simulink library "vmc"  (R2021b)
settings: Solver=VariableStepAuto  StartTime=0.0  StopTime=10.0  RelTol=1e-3
undefined symbols (not defined in the file or in its folder): AVMC_ACCDeltaTqIGain_X_kph, AVMC_ACCDeltaTqIGain_Y_mps2, AVMC_ACCDeltaTqIGainP2_X_kph, AVMC_ACCDeltaTqIGainP2_Y_mps2, AVMC_ACCDeltaTqPGain_X_kph, AVMC_ACCDeltaTqPGain_Y_kph, AVMC_ACCDeltaTqPGainP2_X_kph, AVMC_ACCDeltaTqPGainP2_Y_kph, AVMC_ACCLongSteadyCtrl_X_kph, AVMC_CCAccelCMD_X_kph, AVMC_CCAccelCMD_Y_kph, AVMC_CCDeltaTqIGain_X_kph, AVMC_CCDeltaTqIGain_Y_mps2, AVMC_CCDeltaTqPGain_X_kph, AVMC_CCDeltaTqPGain_Y_kph, AVMC_CCLongSteadyCtrl_X_kph, AVMC_DISCDeltaTqIGainP2_X_kph, AVMC_DISCDeltaTqIGainP2_Y_mps2, AVMC_ESCRegenOut_X_kph, AVMC_ESCRegenOut_Y_Deg, AVMC_ESCRegenOutEnSpd_X_Deg, AVMC_LatESCRegenOut_X_kph, AVMC_LatESCRegenOut_Y_Deg, AVMC_LongAccDeadZone_X_kph, AVMC_LongAccDeadZoneP2_X_kph, AVMC_LongAccFiltTs_X_Gps, AVMC_LongAccFiltTsP2_X_Gps, AVMC_MCPresBaseTq_X_bar, AVMC_MSAAccelCMD_X_kph, AVMC_MSAAccelCMD_Y_kph, AVMC_MSADeltaTqIGain_X_kph, AVMC_MSADeltaTqIGain_Y_mps2, AVMC_MSADeltaTqPGain_X_kph, AVMC_MSADeltaTqPGain_Y_kph, AVMC_MSALongSteadyCtrl_X_kph, AVMC_MSAPedalOvrd_X_kph, AVMC_MSASpdBand_X_kph, AVMC_OPDDisSlideRate_X_Deg, AVMC_RDCDetectTime_X_kph, AVMC_RDCDetectTime_Y_pct, AVMC_RDCEnSlideRate_X_Deg, AVMC_StESCYaw_X_kph, AVMC_StESCYaw_Y_Deg, AVMC_StESCYawCom_X_kph, AVMC_StESCYawCom_Y_Gps, AVMC_TMSpdBaseTq_X_rpm, C_TASK_10MS_S, C_TASK_5MS_S, DEG2RAD, Discrete, ENUM_ADASACCSTA_ACTIVE, ENUM_ADASACCSTA_OVERRIDE, ENUM_ADASACCSTA_STANDBY, ENUM_ADASMSASTA_ACTIVE, ENUM_ADASMSASTA_ERROR, ENUM_ADASMSASTA_OFF, ENUM_ADASMSASTA_OVERSPEED, ENUM_ADASMSASTA_STANDBY, ENUM_ADASMSASTA_UNDERSPEED, ENUM_ADASMSASTA_UNLIMIT ... (+254)
libraries: hcu_lib x57, simulink x49, ctrlSharedLib x6, simulink_extras x1
(part 2 of 9)

== system vmc/VMC/APS function ==
  VTQD_ExternalTqAllow_flg : Inport
  VTQD_ExtShiftAllow_flg : Inport  Port=2
  VTQD_ExtDoorAllow_flg : Inport  Port=3
  VTQD_GearActualPosn_enum : Inport  Port=4
  VINP_APSStaSys_enum : Inport  Port=5
  VINP_APSVMCReqA_flg : Inport  Port=6
  VINP_APSShiftPosnReq_enum : Inport  Port=7
  VINP_APSSpeedCMD_kph : Inport  Port=8
  VINP_CAASVMCReqA_flg : Inport  Port=9
  task_time_s : Inport  Port=10
  BTQD_outputs : Inport  Port=11  OutDataTypeStr=Bus: BTQD_outputs
  VINP_SCPSystemMode_enum : Inport  Port=12
  VVMC_ADASActive_flg : Inport  Port=13
  BINP_APM_outputs : Inport  Port=14  OutDataTypeStr=Bus: BINP_APM_outputs
  VINP_VehSpeed_kph : Inport  Port=15
  VVMC_CruzActive_flg : Inport  Port=16
  VINP_ADASACCSta_enum : Inport  Port=17
  VINP_MCPressure_bar : Inport  Port=18
  VINP_BrkSwSta_flg : Inport  Port=19
  VINP_BrkPedalPos_pct : Inport  Port=20
  VVMC_AllowSetSpd_flg : Inport  Port=21
  AND : Logic  Inputs=4  AllPortsSameDT=off  OutDataTypeStr=boolean
  AND1 : Logic  Operator=OR  AllPortsSameDT=off  OutDataTypeStr=boolean
  AND2 : Logic  Inputs=4  AllPortsSameDT=off  OutDataTypeStr=boolean
  Bus Selector3 : BusSelector  OutputSignals=VTQD_APSDecReqA_flg
  CAAS HandShake : Subsystem
  Command Determination : Subsystem
  Constant1 : Constant  Value=ENUM_ADASACCSTA_ACTIVE
  Constant2 : Constant  Value=ENUM_ADASACCSTA_STANDBY
  Constant3 : Constant  Value=KVMC_APSACCSetTest_flg
  Constant4 : Constant  Value=KVMC_APSAllowSetACCMCP_bar
  Constant5 : Constant  Value=ZERO_FLOAT
  Constant6 : Constant  Value=TRUE
  Constant7 : Constant  Value=KVMC_APSAllowSetACCPosn_pct
  Data Type Conversion : DataTypeConversion  OutDataTypeStr=uint8
  Hand Shake : Subsystem
  NOT : Logic  Operator=NOT  AllPortsSameDT=off  OutDataTypeStr=boolean
  NOT1 : Logic  Operator=NOT  AllPortsSameDT=off  OutDataTypeStr=boolean
  Relational Operator : RelationalOperator  Operator===  OutDataTypeStr=boolean  RndMeth=Simplest
  Relational Operator1 : RelationalOperator  Operator===  OutDataTypeStr=boolean  RndMeth=Simplest
  Relational Operator2 : RelationalOperator  Operator=>  OutDataTypeStr=boolean  RndMeth=Simplest
  Relational Operator3 : RelationalOperator  Operator=>  OutDataTypeStr=boolean  RndMeth=Simplest
  Relational Operator4 : RelationalOperator  Operator=>  OutDataTypeStr=boolean  RndMeth=Simplest
  SR_Latch2 : hcu_lib/Basic_Blocks/SR_Latch
  Signal Rounting : Subsystem
  Switch : Switch  Criteria=u2 > Threshold
  VVMC_APSCtrlAvail_flg : Outport
  VVMC_APSActive_flg : Outport  Port=2
  VVMC_APSSpeedCMD_kph : Outport  Port=3
  VVMC_APSShiftPosnReq_enum : Outport  Port=4
  VVMC_APSStaSys_enum : Outport  Port=5
  VVMC_APSDecReqA_flg : Outport  Port=6
  VVMC_APSDecReq_mps2 : Outport  Port=7
  VVMC_APSReq_enum : Outport  Port=8
  VVMC_CAASCtrlAvail_flg : Outport  Port=9
  VVMC_CAASActive_flg : Outport  Port=10
  wires:
  Command Determination/2(VVMC_APSShiftPosnReq_enum) -> VVMC_APSShiftPosnReq_enum/1
  Command Determination/1(VVMC_APSSpeedCMD_kph) -> VVMC_APSSpeedCMD_kph/1
  [VINP_APSSpeedCMD_kph] -> Command Determination/4(VINP_APSSpeedCMD_kph)
  [VINP_APSShiftPosnReq_enum] -> Command Determination/3(VINP_APSShiftPosnReq_enum)
  [VINP_APSStaSys_enum] -> Command Determination/2(VINP_APSStaSys_enum)
  [VVMC_APSActive_flg] -> Command Determination/1(VVMC_APSActive_flg)
  [VTQD_ExtShiftAllow_flg] -> Hand Shake/3(VTQD_ExtShiftAllow_flg)
  [VTQD_ExternalTqAllow_flg] -> Hand Shake/2(VTQD_ExternalTqAllow_flg)
  [task_time_s] -> Hand Shake/1(task_time_s)
  task_time_s/1 -> [task_time_s]
  VINP_APSSpeedCMD_kph/1 -> [VINP_APSSpeedCMD_kph]
  VINP_APSShiftPosnReq_enum/1 -> [VINP_APSShiftPosnReq_enum]
  VINP_APSVMCReqA_flg/1 -> [VINP_APSVMCReqA_flg]
  VINP_APSStaSys_enum/1 -> [VINP_APSStaSys_enum]
  VVMC_ADASActive_flg/1 -> [VVMC_ADASActive_flg]
  BTQD_outputs/1 -> [BTQD_outputs]
  [VVMC_APSActive_flg] -> Signal Rounting/3(VVMC_APSActive_flg)
  [VVMC_ADASActive_flg] -> Signal Rounting/4(VVMC_ADASActive_flg)
  [BTQD_outputs] -> Signal Rounting/2(BTQD_outputs)
  Signal Rounting/1(VVMC_APSStaSys_enum) -> VVMC_APSStaSys_enum/1
  Signal Rounting/4(VVMC_APSReq_enum) -> VVMC_APSReq_enum/1
  Signal Rounting/3(VVMC_APSDecReq_mps2) -> VVMC_APSDecReq_mps2/1
  Signal Rounting/2(VVMC_APSDecReqA_flg) -> VVMC_APSDecReqA_flg/1
  VTQD_ExtDoorAllow_flg/1 -> [VTQD_ExtDoorAllow_flg]
  VTQD_ExternalTqAllow_flg/1 -> [VTQD_ExternalTqAllow_flg]
  VTQD_ExtShiftAllow_flg/1 -> [VTQD_ExtShiftAllow_flg]
  VINP_SCPSystemMode_enum/1 -> Data Type Conversion/1
  [VTQD_ExtDoorAllow_flg] -> Hand Shake/6(VTQD_ExtDoorAllow_flg)
  [BINP_APM_outputs] -> Signal Rounting/5(BINP_APM_outputs)
  [VINP_APSVMCReqA_flg] -> Hand Shake/4(VINP_APSVMCReqA_flg)
  [VINP_APSStaSys_enum] -> Hand Shake/5(VINP_APSStaSys_enum)
  BINP_APM_outputs/1 -> [BINP_APM_outputs]
  VTQD_GearActualPosn_enum/1 -> [VTQD_GearActualPosn_enum]
  [VINP_SCPSystemMode_enum] -> Signal Rounting/1(VINP_SCPSystemMode_enum)
  [VTQD_GearActualPosn_enum] -> Signal Rounting/6(VTQD_GearActualPosn_enum)
  Data Type Conversion/1 -> [VINP_SCPSystemMode_enum]
  VINP_CAASVMCReqA_flg/1 -> [VINP_CAASVMCReqA_flg]
  [VVMC_CAASActive_flg] -> Signal Rounting/7(VVMC_CAASActive_flg)
  [task_time_s] -> CAAS HandShake/4(task_time_s)
  [VVMC_CruzActive_flg] -> CAAS HandShake/3(VVMC_CruzActive_flg)
  CAAS HandShake/2(VVMC_CAASActive_flg) -> VVMC_CAASActive_flg/1, [VVMC_CAASActive_flg]
  [VINP_VehSpeed_kph] -> CAAS HandShake/1(VINP_VehSpeed_kph)
  [VVMC_ADASActive_flg] -> CAAS HandShake/2(VVMC_ADASActive_flg)
  CAAS HandShake/1(VVMC_CAASCtrlAvail_flg) -> VVMC_CAASCtrlAvail_flg/1
  [VINP_CAASVMCReqA_flg] -> CAAS HandShake/5(VINP_CAASVMCReqA_flg)
  VINP_VehSpeed_kph/1 -> [VINP_VehSpeed_kph]
  VVMC_CruzActive_flg/1 -> [VVMC_CruzActive_flg]
  Hand Shake/1(VVMC_APSCtrlAvail_flg) -> VVMC_APSCtrlAvail_flg/1
  Hand Shake/2(VVMC_APSActive_flg) -> [VVMC_APSActive_flg], VVMC_APSActive_flg/1
  Relational Operator4/1 -> AND2/4
  Constant2/1 -> Relational Operator/2
  VINP_BrkPedalPos_pct/1 -> Relational Operator4/1
  Constant5/1 -> Relational Operator3/2
  [BTQD_outputs] -> Bus Selector3/1
  AND/1 -> SR_Latch2/1
  Relational Operator2/1 -> AND2/2
  Constant6/1 -> Switch/3
  VINP_MCPressure_bar/1 -> Relational Operator2/1
  AND2/1 -> AND/3
  [VINP_BrkSwSta_flg] -> NOT/1
  VINP_BrkSwSta_flg/1 -> [VINP_BrkSwSta_flg], AND2/1
  [VINP_VehSpeed_kph] -> Relational Operator3/1
  Constant3/1 -> AND/4
  NOT1/1 -> AND2/3
  Relational Operator3/1 -> NOT1/1
  SR_Latch2/1 -> Switch/1  "VVMC_SetACCDisableAPS_flg"
  NOT/1 -> AND1/2
  Constant7/1 -> Relational Operator4/2
  VINP_ADASACCSta_enum/1 -> [VINP_ADASACCSta_enum], Relational Operator/1
  Switch/1 -> [VVMC_SetACCDisableAPS_flg]
  Constant1/1 -> Relational Operator1/2
  Constant4/1 -> Relational Operator2/2
  Relational Operator/1 -> AND/1
  Relational Operator1/1 -> AND1/1
  AND1/1 -> SR_Latch2/2
  VVMC_AllowSetSpd_flg/1 -> AND/2
  [VINP_ADASACCSta_enum] -> Relational Operator1/1
  Bus Selector3/1 -> Switch/2  "<VTQD_APSDecReqA_flg>"
  [VVMC_SetACCDisableAPS_flg] -> Signal Rounting/8(VVMC_SetACCDisableAPS_flg)

== system vmc/VMC/CruiseControlFunction ==
  VTQD_ExternalTqAllow_flg : Inport
  VTQD_DriverWhlTqDem_Nm : Inport  Port=2
  VTQD_LowIdleAccPedal_flg : Inport  Port=3
  VTQD_GearActualPosn_enum : Inport  Port=4
  VTQD_ExtDoorAllow_flg : Inport  Port=5
  VINP_ZoneSpdCrlMode_enum : Inport  Port=6
  VINP_SetSpd_kph : Inport  Port=7
  VINP_SWCResUpSta_flg : Inport  Port=8
  VINP_SWCSetdownSta_flg : Inport  Port=9
  VINP_SWCCANCELSta_flg : Inport  Port=10
  VINP_BrakeSWGPIO_flg : Inport  Port=11
  VINP_BrkSwSta_flg : Inport  Port=12
  VINP_VehSpeed_kph : Inport  Port=13
  VINP_BrkPedalPos_pct : Inport  Port=14
  VVMC_LongAcc_Gps : Inport  Port=15
  VVMC_CalMeterSpeed_kph : Inport  Port=16
  CCActiveDetermination : Subsystem
  CCDemandTorqueCalculation : Subsystem
  CCTorqueSourceDetermination : Subsystem
  Data Type Conversion : DataTypeConversion  OutDataTypeStr=uint8
  VVMC_CCCtrlSta_enum : Outport
  VVMC_CCSpdWar_flg : Outport  Port=2
  VVMC_CruzWhlTqReq_N m : Outport  Port=3
  VVMC_CruzActive_flg : Outport  Port=4
  VVMC_CCPedalOvrd_flg : Outport  Port=5
  wires:
  [VVMC_CruzWhlTqReq_Nm] -> VVMC_CruzWhlTqReq_N m/1
  VINP_SWCResUpSta_flg/1 -> [VINP_SWCResUpSta_flg]
  VINP_SWCCANCELSta_flg/1 -> [VINP_SWCCANCELSta_flg]
  VTQD_DriverWhlTqDem_Nm/1 -> [VTQD_DriverWhlTqDem_Nm]
  VINP_ZoneSpdCrlMode_enum/1 -> [VINP_ZoneSpdCrlMode_enum]
  VINP_VehSpeed_kph/1 -> [VINP_VehSpeed_kph]
  VTQD_LowIdleAccPedal_flg/1 -> [VTQD_LowIdleAccPedal_flg]
  [VVMC_CCCtrlSta_enum] -> VVMC_CCCtrlSta_enum/1
  [VVMC_CCSpdWar_flg] -> VVMC_CCSpdWar_flg/1
  [VVMC_CruzActive_flg] -> VVMC_CruzActive_flg/1
  VINP_SWCSetdownSta_flg/1 -> [VINP_SWCSetdownSta_flg]
  VVMC_LongAcc_Gps/1 -> [VVMC_LongAcc_Gps]
  VTQD_ExternalTqAllow_flg/1 -> [VTQD_ExternalTqAllow_flg]
  VINP_BrkSwSta_flg/1 -> [VINP_BrkSwSta_flg]
  VINP_SetSpd_kph/1 -> [VINP_SetSpd_kph]
  [VVMC_CCPedalOvrd_flg] -> VVMC_CCPedalOvrd_flg/1
  VINP_BrakeSWGPIO_flg/1 -> [VINP_BrakeSWGPIO_flg]
  CCTorqueSourceDetermination/2(VVMC_CCPedalOvrd_flg) -> [VVMC_CCPedalOvrd_flg]
  CCTorqueSourceDetermination/1(VVMC_CruzWhlTqReq_Nm) -> [VVMC_CruzWhlTqReq_Nm]
  [VTQD_DriverWhlTqDem_Nm] -> CCTorqueSourceDetermination/1(VTQD_DriverWhlTqDem_Nm)
  [VTQD_LowIdleAccPedal_flg] -> CCTorqueSourceDetermination/4(VTQD_LowIdleAccPedal_flg)
  [VVMC_CruzActive_flg] -> CCTorqueSourceDetermination/3(VVMC_CruzActive_flg)
  [VVMC_CruzWhlTqCal_Nm] -> CCTorqueSourceDetermination/2(VVMC_CruzWhlTqCal_Nm)
  [VINP_VehSpeed_kph] -> CCDemandTorqueCalculation/2(VINP_VehSpeed_kph)
  [VVMC_CCPedalOvrd_flg] -> CCDemandTorqueCalculation/6(VVMC_CCPedalOvrd_flg)
  [VINP_SetSpd_kph] -> CCDemandTorqueCalculation/1(VINP_SetSpd_kph)
  [VVMC_CruzActive_flg] -> CCDemandTorqueCalculation/3(VVMC_CruzActive_flg)
  CCDemandTorqueCalculation/1(VVMC_CruzWhlTqCal_Nm) -> [VVMC_CruzWhlTqCal_Nm]
  [VTQD_DriverWhlTqDem_Nm] -> CCDemandTorqueCalculation/4(VTQD_DriverWhlTqDem_Nm)
  [VVMC_LongAcc_Gps] -> CCDemandTorqueCalculation/5(VVMC_LongAcc_Gps)
  [VINP_SWCSetdownSta_flg] -> CCActiveDetermination/3(VINP_SWCSetdownSta_flg)
  [VINP_SetSpd_kph] -> Data Type Conversion/1
  [VVMC_CCPedalOvrd_flg] -> CCActiveDetermination/10(VVMC_CCPedalOvrd_flg)
  [VINP_SWCCANCELSta_flg] -> CCActiveDetermination/8(VINP_SWCCANCELSta_flg)
  CCActiveDetermination/3(VVMC_CruzActive_flg) -> [VVMC_CruzActive_flg]
  CCActiveDetermination/1(VVMC_CCCtrlSta_enum) -> [VVMC_CCCtrlSta_enum]
  [VTQD_ExternalTqAllow_flg] -> CCActiveDetermination/2(VTQD_ExternalTqAllow_flg)
  [VINP_ZoneSpdCrlMode_enum] -> CCActiveDetermination/1(VINP_ZoneSpdCrlMode_enum)
  [VINP_VehSpeed_kph] -> CCActiveDetermination/5(VINP_VehSpeed_kph)
  [VINP_BrakeSWGPIO_flg] -> CCActiveDetermination/7(VINP_BrakeSWGPIO_flg)
  [VINP_SWCResUpSta_flg] -> CCActiveDetermination/4(VINP_SWCResUpSta_flg)
  [VINP_BrkSwSta_flg] -> CCActiveDetermination/9(VINP_BrkSwSta_flg)
  CCActiveDetermination/2(VVMC_CCSpdWar_flg) -> [VVMC_CCSpdWar_flg]
  VTQD_GearActualPosn_enum/1 -> [VTQD_GearActualPosn_enum]
  [VTQD_GearActualPosn_enum] -> CCActiveDetermination/11(VTQD_GearActualPosn_enum)
  VVMC_CalMeterSpeed_kph/1 -> [VVMC_CalMeterSpeed_kph]
  [VVMC_CalMeterSpeed_kph] -> CCDemandTorqueCalculation/7(VVMC_CalMeterSpeed_kph)
  VINP_BrkPedalPos_pct/1 -> [VINP_BrkPedalPos_pct]
  [VINP_BrkPedalPos_pct] -> CCActiveDetermination/12(VINP_BrkPedalPos_pct)
  Data Type Conversion/1 -> CCActiveDetermination/6(VINP_SetSpd_kph)
  VTQD_ExtDoorAllow_flg/1 -> [VTQD_ExtDoorAllow_flg]
  [VTQD_ExtDoorAllow_flg] -> CCActiveDetermination/13(VTQD_ExtDoorAllow_flg)
  [VVMC_CalMeterSpeed_kph] -> CCActiveDetermination/14(VVMC_CalMeterSpeed_kph)

== system vmc/VMC/IMU ==
  VINP_MemOffsetGyroX_raw16 : Inport
  VINP_MemOffsetGyroY_raw16 : Inport  Port=2
  VINP_MemOffsetGyroZ_raw16 : Inport  Port=3
  VINP_MemOffsetAccX_raw16 : Inport  Port=4
  VINP_MemOffsetAccY_raw16 : Inport  Port=5
  VINP_MemOffsetAccZ_raw16 : Inport  Port=6
  VINP_SensingGyroX_raw16 : Inport  Port=7
  VINP_SensingGyroY_raw16 : Inport  Port=8
  VINP_SensingGyroZ_raw16 : Inport  Port=9
  VINP_SensingAccX_raw16 : Inport  Port=10
  VINP_SensingAccY_raw16 : Inport  Port=11
  VINP_SensingAccZ_raw16 : Inport  Port=12
  task_time_s : Inport  Port=13
  Constant : Constant  Value=KVMC_IMUEnaCmd_flg
  IMU memorized offset result : Subsystem
  "IMU sensing result " : Subsystem
  VVMC_IMUEnaCmd_flg : Outport
  VVMC_CalibratedAccX_G : Outport  Port=2
  VVMC_CalibratedGyroY_Dps : Outport  Port=3
  VVMC_CalibratedAccY_G : Outport  Port=4
  wires:
  VINP_MemOffsetGyroX_raw16/1 -> [VINP_MemOffsetGyroX_raw16]
  VINP_MemOffsetGyroY_raw16/1 -> [VINP_MemOffsetGyroY_raw16]
  VINP_MemOffsetGyroZ_raw16/1 -> [VINP_MemOffsetGyroZ_raw16]
  VINP_MemOffsetAccX_raw16/1 -> [VINP_MemOffsetAccX_raw16]
  VINP_MemOffsetAccY_raw16/1 -> [VINP_MemOffsetAccY_raw16]
  VINP_MemOffsetAccZ_raw16/1 -> [VINP_MemOffsetAccZ_raw16]
  VINP_SensingGyroX_raw16/1 -> [VINP_SensingGyroX_raw16]
  VINP_SensingGyroY_raw16/1 -> [VINP_SensingGyroY_raw16]
  VINP_SensingGyroZ_raw16/1 -> [VINP_SensingGyroZ_raw16]
  VINP_SensingAccX_raw16/1 -> [VINP_SensingAccX_raw16]
  VINP_SensingAccY_raw16/1 -> [VINP_SensingAccY_raw16]
  VINP_SensingAccZ_raw16/1 -> [VINP_SensingAccZ_raw16]
  [VINP_MemOffsetGyroX_raw16] -> IMU memorized offset result/1(VINP_MemOffsetGyroX_raw16)
  [VINP_MemOffsetGyroY_raw16] -> IMU memorized offset result/2(VINP_MemOffsetGyroY_raw16)
  [VINP_MemOffsetGyroZ_raw16] -> IMU memorized offset result/3(VINP_MemOffsetGyroZ_raw16)
  [VINP_MemOffsetAccX_raw16] -> IMU memorized offset result/4(VINP_MemOffsetAccX_raw16)
  [VINP_MemOffsetAccY_raw16] -> IMU memorized offset result/5(VINP_MemOffsetAccY_raw16)
  [VINP_MemOffsetAccZ_raw16] -> IMU memorized offset result/6(VINP_MemOffsetAccZ_raw16)
  IMU memorized offset result/6(VVMC_MemOffsetAccZ_G) -> [VVMC_MemOffsetAccZ_G]
  IMU memorized offset result/5(VVMC_MemOffsetAccY_G) -> [VVMC_MemOffsetAccY_G]
  IMU memorized offset result/4(VVMC_MemOffsetAccX_G) -> [VVMC_MemOffsetAccX_G]
  IMU memorized offset result/3(VVMC_MemOffsetGyroZ_Dps) -> [VVMC_MemOffsetGyroZ_Dps]
  IMU memorized offset result/2(VVMC_MemOffsetGyroY_Dps) -> [VVMC_MemOffsetGyroY_Dps]
  IMU memorized offset result/1(VVMC_MemOffsetGyroX_Dps) -> [VVMC_MemOffsetGyroX_Dps]
  [VVMC_MemOffsetGyroY_Dps] -> "IMU sensing result "/8(VVMC_MemOffsetGyroY_Dps)
  [VVMC_MemOffsetAccX_G] -> "IMU sensing result "/10(VVMC_MemOffsetAccX_G)
  [VVMC_MemOffsetGyroZ_Dps] -> "IMU sensing result "/9(VVMC_MemOffsetGyroZ_Dps)
  [VVMC_MemOffsetAccY_G] -> "IMU sensing result "/11(VVMC_MemOffsetAccY_G)
  [VVMC_MemOffsetGyroX_Dps] -> "IMU sensing result "/7(VVMC_MemOffsetGyroX_Dps)
  [VVMC_MemOffsetAccZ_G] -> "IMU sensing result "/12(VVMC_MemOffsetAccZ_G)
  [VINP_SensingGyroX_raw16] -> "IMU sensing result "/1(VINP_SensingGyroX_raw16)
  [VINP_SensingAccZ_raw16] -> "IMU sensing result "/6(VINP_SensingAccZ_raw16)
  [VINP_SensingAccY_raw16] -> "IMU sensing result "/5(VINP_SensingAccY_raw16)
  [VINP_SensingAccX_raw16] -> "IMU sensing result "/4(VINP_SensingAccX_raw16)
  [VINP_SensingGyroZ_raw16] -> "IMU sensing result "/3(VINP_SensingGyroZ_raw16)
  [VINP_SensingGyroY_raw16] -> "IMU sensing result "/2(VINP_SensingGyroY_raw16)
  Constant/1 -> [VVMC_IMUEnaCmd_flg]  "VVMC_IMUEnaCmd_flg"
  [VVMC_IMUEnaCmd_flg] -> VVMC_IMUEnaCmd_flg/1
  "IMU sensing result "/1(VVMC_CalibratedAccX_G) -> [VVMC_CalibratedAccX_G]
  [VVMC_CalibratedAccX_G] -> VVMC_CalibratedAccX_G/1
  "IMU sensing result "/2(VVMC_CalibratedGyroY_Dps) -> [VVMC_CalibratedGyroY_Dps]
  "IMU sensing result "/3(VVMC_CalibratedAccY_G) -> [VVMC_CalibratedAccY_G]
  [VVMC_CalibratedGyroY_Dps] -> VVMC_CalibratedGyroY_Dps/1
  [VVMC_CalibratedAccY_G] -> VVMC_CalibratedAccY_G/1
  task_time_s/1 -> [task_time_s]
  [task_time_s] -> "IMU sensing result "/13(task_time_s)

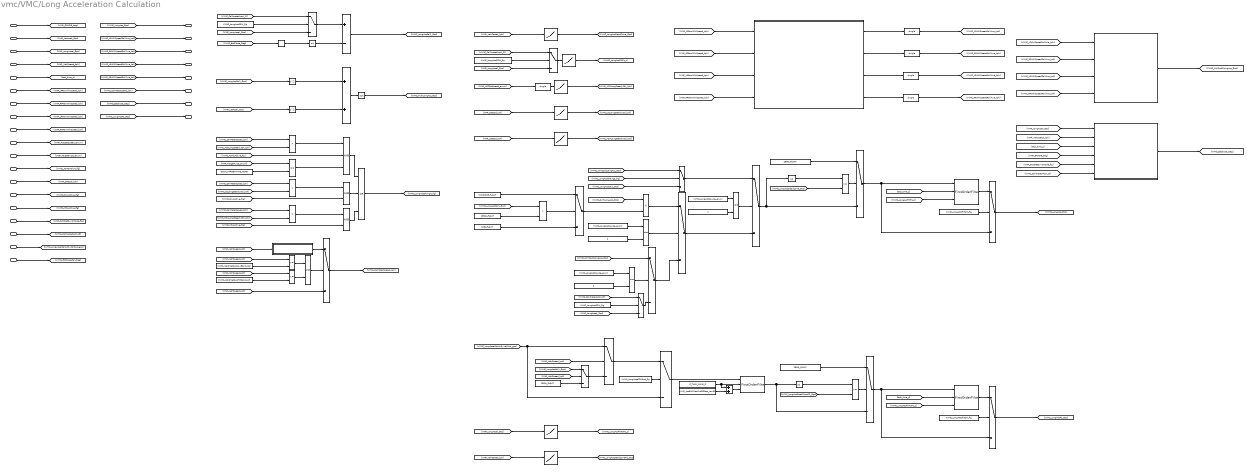
== system vmc/VMC/Long Acceleration Calculation ==
  VINP_GRADE_deg : Inport
  VINP_LatAccel_Gps : Inport  Port=2
  VINP_LongAccel_Gps : Inport  Port=3
  VINP_VehSpeed_kph : Inport  Port=4
  VINP_LFRawWhlSpeed_kph : Inport  Port=5
  VINP_RFRawWhlSpeed_kph : Inport  Port=6
  VINP_LRRawWhlSpeed_kph : Inport  Port=7
  VINP_RRRawWhlSpeed_kph : Inport  Port=8
  VINP_ACCSetSpeed_enum : Inport  Port=9
  VINP_TargetType_enum : Inport  Port=10
  VINP_SetSpd_kph : Inport  Port=11
  VVMC_ADASActive_flg : Inport  Port=12
  VVMC_CruzActive_flg : Inport  Port=13
  task_time_s : Inport  Port=14
  VVMC_MSAActive_flg : Inport  Port=15
  VINP_DIDGetDynoMode_flg : Inport  Port=16
  VVMC_CalibratedAccX_G : Inport  Port=17
  VVMC_LongAccelCalcuByVehSpd_gps : Inport  Port=18
  VVMC_EstSlopeCal_Deg : Inport  Port=19
  AND : Logic  Inputs=3  AllPortsSameDT=off  OutDataTypeStr=boolean
  AND1 : Logic  AllPortsSameDT=off  OutDataTypeStr=boolean
  AND2 : Logic  AllPortsSameDT=off  OutDataTypeStr=boolean
  AND3 : Logic  AllPortsSameDT=off  OutDataTypeStr=boolean
  Abs : Abs
  Abs1 : Abs
  Add : Sum  Inputs=+-
  Add1 : Sum
  Add9 : Sum
  Cast To Single{,1..3} (4 alike) : DataTypeConversion  OutDataTypeStr=single
  Constant{,7,17,19} (4 alike) : Constant  Value=ZERO_FLOAT
  Constant1 : Constant  Value=MINUSONE_FLOAT
  Constant10 : Constant  Value=3  OutDataTypeStr=uint8
  Constant11 : Constant  Value=KVMC_Veh2MetSpdLowBand_kph
  Constant12 : Constant  Value=ENUM_TARGETTYPE_NONE
  Constant13 : Constant  Value=KVMC_Veh2MetSpdHiBand_kph
  Constant14 : Constant  Value=KVMC_LongAccGSW_flg
  Constant15 : Constant  Value=KVMC_LongAccGSW_flg
  Constant16 : Constant  Value=KVMC_LongAccGSW_flg
  Constant18 : Constant  Value=KVMC_LongACCFiltSW_flg
  Constant2 : Constant  Value=ONE_FLOAT
  Constant27 : Constant  Value=KVMC_AccBWFilterCutOffFreq_raw32
  Constant29 : Constant  Value=C_TASK_10MS_S
  Constant3 : Constant  Value=KVMC_LongAccSource_enum
  Constant30 : Constant  Value=KVMC_LongAccelSWSpd_flg
  Constant4 : Constant  Value=2  OutDataTypeStr=uint8
  Constant5 : Constant  Value=KVMC_LongAccSource_enum
  Constant6 : Constant  OutDataTypeStr=uint8
  Constant8 : Constant  Value=KVMC_LongACCFiltSW_flg
  Constant9 : Constant  Value=KVMC_LongAccSource_enum
  Data Type Conversion : DataTypeConversion  OutDataTypeStr=single
  Degrees to Radians : simulink_extras/Transformations/Degrees to Radians
  Equal : RelationalOperator  Operator===  OutDataTypeStr=boolean  RndMeth=Simplest
  Equal1 : RelationalOperator  Operator===  OutDataTypeStr=boolean  RndMeth=Simplest
  Equal2 : RelationalOperator  Operator===  OutDataTypeStr=boolean  RndMeth=Simplest
  Estimate Slope : Subsystem
  FirstOrderFilter : hcu_lib/Basic_Blocks/FirstOrderFilter
  FirstOrderFilter1 : hcu_lib/Basic_Blocks/FirstOrderFilter
  FirstOrderFilter8 : hcu_lib/Basic_Blocks/FirstOrderFilter
  MVMC_ACCLongSteadyCtrl_Y_kph : Lookup_n-D  NumberOfTableDimensions=1  BreakpointsForDimension1=AVMC_ACCLongSteadyCtrl_X_kph  Table=MVMC_ACCLongSteadyCtrl_Y_kph  ExtrapMethod=Clip  InternalRulePriority=Speed  RndMeth=Simplest  InputSameDT=on
  MVMC_CCLongSteadyCtrl_Y_kph : Lookup_n-D  NumberOfTableDimensions=1  BreakpointsForDimension1=AVMC_CCLongSteadyCtrl_X_kph  Table=MVMC_CCLongSteadyCtrl_Y_kph  ExtrapMethod=Clip  InternalRulePriority=Speed  RndMeth=Simplest  InputSameDT=on
  MVMC_LongAccDeadZoneP2_Y_Gps : Lookup_n-D  NumberOfTableDimensions=1  BreakpointsForDimension1=AVMC_LongAccDeadZoneP2_X_kph  Table=MVMC_LongAccDeadZoneP2_Y_Gps  ExtrapMethod=Clip  InternalRulePriority=Speed  RndMeth=Simplest  InputSameDT=on
  MVMC_LongAccDeadZone_Y_Gps : Lookup_n-D  NumberOfTableDimensions=1  BreakpointsForDimension1=AVMC_LongAccDeadZone_X_kph  Table=MVMC_LongAccDeadZone_Y_Gps  ExtrapMethod=Clip  InternalRulePriority=Speed  RndMeth=Simplest  InputSameDT=on
  MVMC_LongAccFiltTsP2_Y_c : Lookup_n-D  NumberOfTableDimensions=1  BreakpointsForDimension1=AVMC_LongAccFiltTsP2_X_Gps  Table=MVMC_LongAccFiltTsP2_Y_c  ExtrapMethod=Clip  InternalRulePriority=Speed  RndMeth=Simplest  InputSameDT=on
  MVMC_LongAccFiltTs_Y_c : Lookup_n-D  NumberOfTableDimensions=1  BreakpointsForDimension1=AVMC_LongAccFiltTs_X_Gps  Table=MVMC_LongAccFiltTs_Y_c  ExtrapMethod=Clip  InternalRulePriority=Speed  RndMeth=Simplest  InputSameDT=on
  MVMC_MSALongSteadyCtrl_Y_kph : Lookup_n-D  NumberOfTableDimensions=1  BreakpointsForDimension1=AVMC_MSALongSteadyCtrl_X_kph  Table=MVMC_MSALongSteadyCtrl_Y_kph  ExtrapMethod=Clip  InternalRulePriority=Speed  RndMeth=Simplest  InputSameDT=on
  Math Function1 : Math  Operator=square  SaturateOnIntegerOverflow=on
  Math Function2 : Math  Operator=square  SaturateOnIntegerOverflow=on
  OR : Logic  Operator=OR  Inputs=3  AllPortsSameDT=off  OutDataTypeStr=boolean
  Product : Product
  Relational Operator : RelationalOperator  Operator=<  OutDataTypeStr=boolean  RndMeth=Simplest
  Relational Operator1 : RelationalOperator  Operator=<=  OutDataTypeStr=boolean  RndMeth=Simplest
  Relational Operator2 : RelationalOperator  Operator=>  OutDataTypeStr=boolean  RndMeth=Simplest
  Relational Operator3 : RelationalOperator  Operator===  OutDataTypeStr=boolean  RndMeth=Simplest
  Relational Operator4 : RelationalOperator  Operator=>  OutDataTypeStr=boolean  RndMeth=Simplest
  Relational Operator5 : RelationalOperator  OutDataTypeStr=boolean  RndMeth=Simplest
  Relational Operator6 : RelationalOperator  Operator=<=  OutDataTypeStr=boolean  RndMeth=Simplest
  Relational Operator7 : RelationalOperator  Operator=>  OutDataTypeStr=boolean  RndMeth=Simplest
  Relational Operator8 : RelationalOperator  Operator=<=  OutDataTypeStr=boolean  RndMeth=Simplest
  Sin : Trigonometry
  Square Root : Sqrt  SaturateOnIntegerOverflow=on
  Switch{,1..11,13..15} (15 alike) : Switch  Criteria=u2 > Threshold
  Switch12 : Switch  Criteria=u2 > Threshold  Threshold=KVMC_LongAccelSWSpd_kph
  Vehicle to Meter Speed : Subsystem
  Wheel speed to long accelerate calculation : Subsystem
  WheelSpeedRollingAverage : Subsystem
  VVMC_LongAcc_Gps : Outport
  VVMC_LFWhlSpeedRollAve_kph : Outport  Port=2
  VVMC_RFWhlSpeedRollAve_kph : Outport  Port=3
  VVMC_LRWhlSpeedRollAve_kph : Outport  Port=4
  VVMC_RRWhlSpeedRollAve_kph : Outport  Port=5
  VVMC_CalMeterSpeed_kph : Outport  Port=6
  VVMC_EstSlope_Deg : Outport  Port=7
  VVMC_LongAccP2_Gps : Outport  Port=8
  wires:
  [VVMC_LongAcc_Gps] -> VVMC_LongAcc_Gps/1
  Equal1/1 -> Switch2/2
  Constant5/1 -> Equal1/1
  Constant6/1 -> Equal1/2
  Switch1/1 -> Switch2/3
  Constant4/1 -> Equal/2
  Constant3/1 -> Equal/1
  Equal/1 -> Switch1/2
  Product/1 -> Switch1/1  "VVMC_LongAccCal2_Gps"
  [VVMC_PythLongAcc_Gps] -> Product/1
  Switch/1 -> Product/2
  Constant2/1 -> Switch/3
  Constant1/1 -> Switch/1
  Relational Operator/1 -> Switch/2  "VVMC_LongAccNeg_flg"
  Constant/1 -> Relational Operator/2
  [VVMC_LongAccCal1_Gps] -> Relational Operator/1
  Sin/1 -> Add/2  "VVMC_SineGRADE_Gps"
  [VVMC_LongAccCal1_Gps] -> Math Function2/1
  Square Root/1 -> [VVMC_PythLongAcc_Gps]  "VVMC_PythLongAcc_Gps"
  Add1/1 -> Square Root/1
  Math Function2/1 -> Add1/1
  Math Function1/1 -> Add1/2
  [VINP_LatAccel_Gps] -> Math Function1/1
  Add/1 -> [VVMC_LongAccCal1_Gps]  "VVMC_LongAccCal1_Gps"
  Degrees to Radians/1 -> Sin/1  "VVMC_GRADE_rad"
  [VVMC_EstSlope_Deg] -> Degrees to Radians/1
  VINP_LongAccel_Gps/1 -> [VINP_LongAccel_Gps]
  VINP_LatAccel_Gps/1 -> [VINP_LatAccel_Gps]
  VINP_GRADE_deg/1 -> [VINP_GRADE_deg]
  Constant7/1 -> Switch3/1
  [VVMC_LongAccDeadZone_Gps] -> Relational Operator1/2
  Abs/1 -> Relational Operator1/1
  Relational Operator1/1 -> Switch3/2
  Switch2/1 -> Abs/1, Switch3/3
  VINP_VehSpeed_kph/1 -> [VINP_VehSpeed_kph]
  [VINP_VehSpeed_kph] -> MVMC_LongAccDeadZone_Y_Gps/1
  MVMC_LongAccDeadZone_Y_Gps/1 -> [VVMC_LongAccDeadZone_Gps]  "VVMC_LongAccDeadZone_Gps"
  Switch3/1 -> Switch4/3, FirstOrderFilter/1  "VVMC_LongAccTemp_Gps"
  Switch4/1 -> [VVMC_LongAcc_Gps]  "VVMC_LongAcc_Gps"
  FirstOrderFilter/1 -> Switch4/1
  task_time_s/1 -> [task_time_s]
  [task_time_s] -> FirstOrderFilter/2
  Constant8/1 -> Switch4/2
  MVMC_LongAccFiltTs_Y_c/1 -> [VVMC_LongAccFiltTs_c]  "VVMC_LongAccFiltTs_c"
  [VVMC_LongAccFiltTs_c] -> FirstOrderFilter/3
  VINP_LFRawWhlSpeed_kph/1 -> [VINP_LFRawWhlSpeed_kph]
  VINP_RFRawWhlSpeed_kph/1 -> [VINP_RFRawWhlSpeed_kph]
  VINP_LRRawWhlSpeed_kph/1 -> [VINP_LRRawWhlSpeed_kph]
  VINP_RRRawWhlSpeed_kph/1 -> [VINP_RRRawWhlSpeed_kph]
  [VVMC_LFWhlSpeedRollAve_kph] -> Wheel speed to long accelerate calculation/1(VVMC_LFWhlSpeedRollAve_kph)
  [VVMC_RFWhlSpeedRollAve_kph] -> Wheel speed to long accelerate calculation/2(VVMC_RFWhlSpeedRollAve_kph)
  [VVMC_LRWhlSpeedRollAve_kph] -> Wheel speed to long accelerate calculation/3(VVMC_LRWhlSpeedRollAve_kph)
  [VVMC_RRWhlSpeedRollAve_kph] -> Wheel speed to long accelerate calculation/4(VVMC_RRWhlSpeedRollAve_kph)
  [VVMC_LFWhlSpeedRollAve_kph] -> VVMC_LFWhlSpeedRollAve_kph/1
  [VVMC_RFWhlSpeedRollAve_kph] -> VVMC_RFWhlSpeedRollAve_kph/1
  [VVMC_LRWhlSpeedRollAve_kph] -> VVMC_LRWhlSpeedRollAve_kph/1
  [VVMC_RRWhlSpeedRollAve_kph] -> VVMC_RRWhlSpeedRollAve_kph/1
  Wheel speed to long accelerate calculation/1(VVMC_WhlSpd2LongAcc_Gps) -> [VVMC_WhlSpd2LongAcc_Gps]
  Switch5/1 -> Switch1/3
  [VVMC_WhlSpd2LongAcc_Gps] -> Switch5/1
  Equal2/1 -> Switch5/2
  Constant9/1 -> Equal2/1
  Constant10/1 -> Equal2/2
  [VINP_LRRawWhlSpeed_kph] -> WheelSpeedRollingAverage/3(VINP_LRRawWhlSpeed_kph)
  Cast To Single2/1 -> [VVMC_LRWhlSpeedRollAve_kph]  "VVMC_LRWhlSpeedRollAve_kph"
  [VINP_RFRawWhlSpeed_kph] -> WheelSpeedRollingAverage/2(VINP_RFRawWhlSpeed_kph)
  WheelSpeedRollingAverage/2(VVMC_RFWhlSpeedRollAve_kph) -> Cast To Single1/1
  Cast To Single/1 -> [VVMC_LFWhlSpeedRollAve_kph]  "VVMC_LFWhlSpeedRollAve_kph"
  [VINP_RRRawWhlSpeed_kph] -> WheelSpeedRollingAverage/4(VINP_RRRawWhlSpeed_kph)
  WheelSpeedRollingAverage/3(VVMC_LRWhlSpeedRollAve_kph) -> Cast To Single2/1
  WheelSpeedRollingAverage/4(VVMC_RRWhlSpeedRollAve_kph) -> Cast To Single3/1
  Cast To Single3/1 -> [VVMC_RRWhlSpeedRollAve_kph]  "VVMC_RRWhlSpeedRollAve_kph"
  Cast To Single1/1 -> [VVMC_RFWhlSpeedRollAve_kph]  "VVMC_RFWhlSpeedRollAve_kph"
  [VINP_LFRawWhlSpeed_kph] -> WheelSpeedRollingAverage/1(VINP_LFRawWhlSpeed_kph)
  WheelSpeedRollingAverage/1(VVMC_LFWhlSpeedRollAve_kph) -> Cast To Single/1
  [VVMC_LongAccCal1_Gps] -> Switch6/3
  Switch6/1 -> Switch2/1  "VVMC_ActLongAccSource1_Gps"
  [VVMC_WhlSpd2LongAcc_Gps] -> Switch6/1
  [VVMC_CalMeterSpeed_kph] -> Relational Operator2/1
  [VVMC_ACCLongSteadyCtrl_kph] -> Relational Operator2/2
  Constant12/1 -> Relational Operator3/2
  [VINP_TargetType_enum] -> Relational Operator3/1
  Data Type Conversion/1 -> MVMC_ACCLongSteadyCtrl_Y_kph/1
  [VINP_ACCSetSpeed_enum] -> Data Type Conversion/1
  MVMC_ACCLongSteadyCtrl_Y_kph/1 -> [VVMC_ACCLongSteadyCtrl_kph]  "VVMC_ACCLongSteadyCtrl_kph"
  Relational Operator2/1 -> AND/1
  Relational Operator3/1 -> AND/3
  [VVMC_ADASActive_flg] -> AND/2
  MVMC_CCLongSteadyCtrl_Y_kph/1 -> [VVMC_CCLongSteadyCtrl_kph]  "VVMC_CCLongSteadyCtrl_kph"
  [VINP_SetSpd_kph] -> MVMC_CCLongSteadyCtrl_Y_kph/1
  [VVMC_CalMeterSpeed_kph] -> Relational Operator4/1
  Relational Operator4/1 -> AND1/1
  OR/1 -> [VVMC_LongAccChange_flg]  "VVMC_LongAccChange_flg"
  [VVMC_LongAccChange_flg] -> Switch6/2
  VINP_ACCSetSpeed_enum/1 -> [VINP_ACCSetSpeed_enum]
  VINP_TargetType_enum/1 -> [VINP_TargetType_enum]
  VVMC_ADASActive_flg/1 -> [VVMC_ADASActive_flg]
  VINP_SetSpd_kph/1 -> [VINP_SetSpd_kph]
  VVMC_CruzActive_flg/1 -> [VVMC_CruzActive_flg]
  [VINP_VehSpeed_kph] -> Relational Operator5/1
  Constant11/1 -> Relational Operator5/2
  Relational Operator5/1 -> AND2/1
  Relational Operator6/1 -> AND2/2
  Constant13/1 -> Relational Operator6/2
  [VINP_VehSpeed_kph] -> Relational Operator6/1
  AND2/1 -> Switch7/2
  [VINP_VehSpeed_kph] -> Switch7/3
  [VINP_VehSpeed_kph] -> Vehicle to Meter Speed/1(InputSpeed)
  Vehicle to Meter Speed/1(OutputSpeed) -> Switch7/1
  Switch7/1 -> [VVMC_CalMeterSpeed_kph]  "VVMC_CalMeterSpeed_kph"
  [VVMC_CalMeterSpeed_kph] -> VVMC_CalMeterSpeed_kph/1
  [VVMC_MSAActive_flg] -> AND3/2
  Relational Operator7/1 -> AND3/1
  [VVMC_CalMeterSpeed_kph] -> Relational Operator7/1
  AND1/1 -> OR/2
  AND3/1 -> OR/3
  AND/1 -> OR/1
  VVMC_MSAActive_flg/1 -> [VVMC_MSAActive_flg]
  [VINP_SetSpd_kph] -> MVMC_MSALongSteadyCtrl_Y_kph/1
  MVMC_MSALongSteadyCtrl_Y_kph/1 -> [VVMC_MSALongSteadyCtrl_kph]  "VVMC_MSALongSteadyCtrl_kph"
  [VVMC_MSALongSteadyCtrl_kph] -> Relational Operator7/2
  [VINP_VehSpeed_kph] -> Estimate Slope/2(VINP_VehSpeed_kph)
  [VINP_LongAccel_Gps] -> Estimate Slope/1(VINP_LongAccel_Gps)
  [task_time_s] -> Estimate Slope/3(task_time_s)
  [VINP_GRADE_deg] -> Estimate Slope/4(VINP_GRADE_deg)
  Estimate Slope/1(VVMC_EstSlope_Deg) -> [VVMC_EstSlope_Deg]
  [VVMC_EstSlope_Deg] -> VVMC_EstSlope_Deg/1
  [VVMC_CruzActive_flg] -> AND1/2
  [VVMC_CCLongSteadyCtrl_kph] -> Relational Operator4/2
  VINP_DIDGetDynoMode_flg/1 -> [VINP_DIDGetDynoMode_flg]
  [VINP_DIDGetDynoMode_flg] -> Estimate Slope/5(VINP_DIDGetDynoMode_flg)
  VVMC_CalibratedAccX_G/1 -> [VVMC_CalibratedAccX_G]
  [VVMC_CalibratedAccX_G] -> Estimate Slope/6(VVMC_CalibratedAccX_G)
  Switch8/1 -> Add/1
  [VINP_LongAccel_Gps] -> Switch8/3
  [VVMC_CalibratedAccX_G] -> Switch8/1
  Constant14/1 -> Switch8/2
  Constant15/1 -> Switch9/2
  [VVMC_CalibratedAccX_G] -> Switch9/1
  Switch9/1 -> MVMC_LongAccFiltTs_Y_c/1
  [VINP_LongAccel_Gps] -> Switch9/3
  Constant16/1 -> Switch10/2
  [VVMC_CalibratedAccX_G] -> Switch10/1
  Switch10/1 -> Switch5/3
  [VINP_LongAccel_Gps] -> Switch10/3
  Switch13/1 -> [VVMC_LongAccP2_Gps]  "VVMC_LongAccP2_Gps"
  Switch12/1 -> Switch11/1
  Switch11/1 -> FirstOrderFilter8/1
  [VVMC_LongAccDeadZoneP2_Gps] -> Relational Operator8/2
  [VINP_LongAccel_Gps] -> MVMC_LongAccFiltTsP2_Y_c/1
  Constant19/1 -> Switch14/1
  [VVMC_LongAccFiltTsP2_c] -> FirstOrderFilter1/3
  [VINP_VehSpeed_kph] -> Switch12/2
  MVMC_LongAccDeadZoneP2_Y_Gps/1 -> [VVMC_LongAccDeadZoneP2_Gps]  "VVMC_LongAccDeadZoneP2_Gps"
  Add9/1 -> FirstOrderFilter8/3
  Constant29/1 -> Add9/1, FirstOrderFilter8/2
  Relational Operator8/1 -> Switch14/2
  Abs1/1 -> Relational Operator8/1
  Switch15/1 -> Switch12/3
  Constant17/1 -> Switch15/3
  FirstOrderFilter8/1 -> Abs1/1, Switch14/3  "VVMC_LongAccelCalcuByVehSpd_gps"
  MVMC_LongAccFiltTsP2_Y_c/1 -> [VVMC_LongAccFiltTsP2_c]  "VVMC_LongAccFiltTsP2_c"
  [task_time_s] -> FirstOrderFilter1/2
  [VVMC_LongAccCal1_Gps] -> Switch15/1
  [VVMC_LongAccelCalcuByVehSpd_gps] -> Switch12/1, Switch11/3
  FirstOrderFilter1/1 -> Switch13/1
  Constant30/1 -> Switch11/2
  Constant18/1 -> Switch13/2
  Constant27/1 -> Add9/2
  [VINP_VehSpeed_kph] -> MVMC_LongAccDeadZoneP2_Y_Gps/1
  [VINP_VehSpeed_kph] -> Switch15/2
  Switch14/1 -> FirstOrderFilter1/1, Switch13/3
  VVMC_LongAccelCalcuByVehSpd_gps/1 -> [VVMC_LongAccelCalcuByVehSpd_gps]
  VVMC_EstSlopeCal_Deg/1 -> [VVMC_EstSlopeCal_Deg]
  [VVMC_LongAccP2_Gps] -> VVMC_LongAccP2_Gps/1

== system vmc/VMC/LongAccel_EstSlope ==
  VINP_VehSpeed_kph : Inport
  VINP_LongAccel_Gps : Inport  Port=2
  VINP_GRADE_deg : Inport  Port=3
  function : TriggerPort  TriggerType=function-call  VariantControl=(inherit)
  Add2 : Sum
  Add8 : Sum
  Cast To Single8 : DataTypeConversion  OutDataTypeStr=single
  Constant22 : Constant  Value=C_TASK_10MS_S
  Constant23 : Constant  Value=KVMC_VehSpdBWFilter_raw32
  Constant24 : Constant  Value=GRAVITY_G
  Constant25 : Constant  Value=KPH2MPS
  Constant26 : Constant  Value=C_TASK_10MS_S
  Constant5 : Constant  Value=KVMC_RollAveEnTime_s
  Constant6 : Constant  Value=C_TASK_10MS_S
  Divide2 : Product  Inputs=**
  Divide4 : Product  Inputs=*/
  Estimate Slope : Subsystem
  FirstOrderFilter6 : hcu_lib/Basic_Blocks/FirstOrderFilter
  Min1 : MinMax  Inputs=2
  Relational Operator : RelationalOperator  OutDataTypeStr=boolean  RndMeth=Simplest
  VehSpdRollingAverage : Subsystem
  derivative1 : hcu_lib/Basic_Blocks/derivative
  initial: 0 : UnitDelay  SampleTime=-1  HasFrameUpgradeWarning=on
  u2 > 0 (1)6 : Switch  Criteria=u2 > Threshold
  VVMC_EstSlope_Deg : Outport
  VVMC_LongAccelCalcuByVehSpd_gps : Outport  Port=2
  wires:
  VINP_VehSpeed_kph/1 -> [VINP_VehSpeed_kph]
  initial: 0/1 -> Add2/1
  Constant5/1 -> Min1/2, Relational Operator/2
  Constant6/1 -> Add2/2
  Add2/1 -> Min1/1
  Relational Operator/1 -> [VVMC_RollAveEn_flg]
  [VINP_LongAccel_Gps] -> Estimate Slope/1(VINP_LongAccel_Gps)
  [VINP_GRADE_deg] -> Estimate Slope/3(VINP_GRADE_deg)
  [VINP_VehSpeed_kph] -> Estimate Slope/2(VINP_VehSpeed_kph)
  Estimate Slope/1(VVMC_EstSlope_Deg) -> [VVMC_EstSlopeCal_Deg]
  VINP_LongAccel_Gps/1 -> [VINP_LongAccel_Gps]
  VINP_GRADE_deg/1 -> [VINP_GRADE_deg]
  [VVMC_EstSlopeCal_Deg] -> VVMC_EstSlope_Deg/1
  [VINP_VehSpeed_kph] -> VehSpdRollingAverage/1(VINP_VehSpeed_kph)
  Add8/1 -> FirstOrderFilter6/3
  Constant23/1 -> Add8/2
  Constant22/1 -> Add8/1, FirstOrderFilter6/2
  Cast To Single8/1 -> u2 > 0 (1)6/1
  u2 > 0 (1)6/1 -> FirstOrderFilter6/1
  [VINP_VehSpeed_kph] -> u2 > 0 (1)6/3
  [VVMC_RollAveEn_flg] -> u2 > 0 (1)6/2
  FirstOrderFilter6/1 -> [VVMC_VehSpdRollAve_kph]  "VVMC_VehSpdRollAve_kph"
  VehSpdRollingAverage/1(VVMC_VehSpdRollAve_kph) -> Cast To Single8/1
  Constant26/1 -> derivative1/2
  derivative1/1 -> Divide4/1
  Constant24/1 -> Divide4/2
  Constant25/1 -> Divide2/2
  [VVMC_VehSpdRollAve_kph] -> Divide2/1
  Divide2/1 -> derivative1/1
  Divide4/1 -> [VVMC_LongAccelCalcuByVehSpd_gps]  "VVMC_LongAccelCalcuByVehSpd_gps"
  [VVMC_LongAccelCalcuByVehSpd_gps] -> VVMC_LongAccelCalcuByVehSpd_gps/1  "VVMC_LongAccelCalcuByVehSpd_gps"
  Min1/1 -> initial: 0/1, Relational Operator/1

== system vmc/VMC/MSA function ==
  VTQD_ExternalTqAllow_flg : Inport
  VTQD_DriverWhlTqDem_Nm : Inport  Port=2
  VTQD_GearActualPosn_enum : Inport  Port=3
  VINP_ZoneSpdCrlMode_enum : Inport  Port=4
  VINP_SetSpd_kph : Inport  Port=5
  VINP_SWCCANCELSta_flg : Inport  Port=6
  VINP_SWCResUpSta_flg : Inport  Port=7
  VINP_SWCSetdownSta_flg : Inport  Port=8
  VINP_VehSpeed_kph : Inport  Port=9
  VVMC_LongAcc_Gps : Inport  Port=10
  task_time_s : Inport  Port=11
  VDHP_ActAPSPosn_pct : Inport  Port=12
  VVMC_CalMeterSpeed_kph : Inport  Port=13
  VINP_HoodSW_flg : Inport  Port=14
  Anti-Speed Limitation : Subsystem
  Constant6 : Constant  Value=ENUM_EXTRAMSACTRLSTA_ANTISPEEDLIMIT
  Constant7 : Constant  Value=ENUM_EXTRAMSACTRLSTA_OFF
  MSAActivationHandshake : Subsystem
  MSADemandTorqueCalculation : Subsystem
  MSATorqueSourceDetermination : Subsystem
  Switch5 : Switch  Criteria=u2 > Threshold
  VVMC_MSACtrlSta_enum : Outport
  VVMC_MSAWhlTqReq_Nm : Outport  Port=2
  VVMC_MSASpdWar_flg : Outport  Port=3
  VVMC_MSAActive_flg : Outport  Port=4
  VVMC_ExtraMSACtrlSta_enum : Outport  Port=5
  wires:
  MSADemandTorqueCalculation/1(VVMC_MSAWhlTqCal_Nm) -> [VVMC_MSAWhlTqCal_Nm]
  [VVMC_MSASetSpd_kph] -> MSADemandTorqueCalculation/1(VVMC_MSASetSpd_kph)
  [VTQD_DriverWhlTqDem_Nm] -> MSADemandTorqueCalculation/3(VTQD_DriverWhlTqDem_Nm)
  [VVMC_LongAcc_Gps] -> MSADemandTorqueCalculation/4(VVMC_LongAcc_Gps)
  [VVMC_MSAActive_flg] -> MSADemandTorqueCalculation/2(VVMC_MSAActive_flg)
  [VVMC_MSASpdCtrlMode_enum] -> MSAActivationHandshake/1(VVMC_MSASpdCtrlMode_enum)
  MSAActivationHandshake/1(VVMC_MSACtrlSta_enum) -> [VVMC_MSACtrlSta_enum]
  MSAActivationHandshake/2(VVMC_MSASpdWar_flg) -> [VVMC_MSASpdWar_flg]
  MSAActivationHandshake/3(VVMC_MSAActive_flg) -> [VVMC_MSAActive_flg]
  [VVMC_MSACtrlSta_enum] -> VVMC_MSACtrlSta_enum/1
  VINP_ZoneSpdCrlMode_enum/1 -> [VINP_ZoneSpdCrlMode_enum]
  [VVMC_MSAWhlTqReq_Nm] -> VVMC_MSAWhlTqReq_Nm/1
  VINP_SWCCANCELSta_flg/1 -> [VINP_SWCCANCELSta_flg]
  VINP_VehSpeed_kph/1 -> [VINP_VehSpeed_kph]
  [VVMC_MSASpdWar_flg] -> VVMC_MSASpdWar_flg/1
  VTQD_DriverWhlTqDem_Nm/1 -> [VTQD_DriverWhlTqDem_Nm]
  [VVMC_MSAActive_flg] -> VVMC_MSAActive_flg/1
  VTQD_ExternalTqAllow_flg/1 -> [VTQD_ExternalTqAllow_flg]
  VINP_SetSpd_kph/1 -> [VINP_SetSpd_kph]  "VINP_SetSpd_kph"
  VVMC_LongAcc_Gps/1 -> [VVMC_LongAcc_Gps]
  [VVMC_MSAWhlTqCal_Nm] -> MSATorqueSourceDetermination/1(VVMC_MSAWhlTqCal_Nm)
  MSATorqueSourceDetermination/1(VVMC_MSAWhlTqReq_Nm) -> [VVMC_MSAWhlTqReq_Nm]
  [VTQD_DriverWhlTqDem_Nm] -> MSATorqueSourceDetermination/2(VTQD_DriverWhlTqDem_Nm)
  task_time_s/1 -> [task_time_s]
  VTQD_GearActualPosn_enum/1 -> [VTQD_GearActualPosn_enum]
  [VTQD_ExternalTqAllow_flg] -> MSAActivationHandshake/2(VTQD_ExternalTqAllow_flg)
  [VINP_VehSpeed_kph] -> MSAActivationHandshake/3(VINP_VehSpeed_kph)
  [VVMC_MSASetSpd_kph] -> MSAActivationHandshake/4(VVMC_MSASetSpd_kph)
  [VINP_SWCCANCELSta_flg] -> MSAActivationHandshake/5(VINP_SWCCANCELSta_flg)
  [VVMC_MSAUnLimit_flg] -> MSAActivationHandshake/6(VVMC_MSAUnLimit_flg)
  [VTQD_GearActualPosn_enum] -> MSAActivationHandshake/7(VTQD_GearActualPosn_enum)
  [VVMC_MSACtrlSta_enum] -> MSATorqueSourceDetermination/3(VVMC_MSACtrlSta_enum)
  [VVMC_MSAActive_flg] -> MSATorqueSourceDetermination/4(VVMC_MSAActive_flg)
  [VINP_VehSpeed_kph] -> MSATorqueSourceDetermination/5(VINP_VehSpeed_kph)
  [VVMC_MSASetSpd_kph] -> MSATorqueSourceDetermination/6(VVMC_MSASetSpd_kph)
  [task_time_s] -> MSATorqueSourceDetermination/7(task_time_s)
  MSATorqueSourceDetermination/2(VVMC_MSAUnLimit_flg) -> [VVMC_MSAUnLimit_flg]
  VDHP_ActAPSPosn_pct/1 -> [VDHP_ActAPSPosn_pct]
  [VDHP_ActAPSPosn_pct] -> MSATorqueSourceDetermination/8(VDHP_ActAPSPosn_pct)
  [VVMC_MSAUnLimit_flg] -> MSADemandTorqueCalculation/5(VVMC_MSAUnLimit_flg)
  VVMC_CalMeterSpeed_kph/1 -> [VVMC_CalMeterSpeed_kph]
  [VVMC_CalMeterSpeed_kph] -> MSADemandTorqueCalculation/6(VVMC_CalMeterSpeed_kph)
  VINP_SWCResUpSta_flg/1 -> [VINP_SWCResUpSta_flg]
  VINP_SWCSetdownSta_flg/1 -> [VINP_SWCSetdownSta_flg]
  [VINP_SWCResUpSta_flg] -> MSAActivationHandshake/8(VINP_SWCResUpSta_flg)
  [VINP_SWCSetdownSta_flg] -> MSAActivationHandshake/9(VINP_SWCSetdownSta_flg)
  VINP_HoodSW_flg/1 -> [VINP_HoodSW_flg]
  Anti-Speed Limitation/1(VVMC_AntiSpdLimEn_flg) -> [VVMC_AntiSpdLimEn_flg]
  [VINP_HoodSW_flg] -> Anti-Speed Limitation/1(VINP_HoodSW_flg)
  [VINP_SetSpd_kph] -> Anti-Speed Limitation/4(VINP_SetSpd_kph)
  [VINP_ZoneSpdCrlMode_enum] -> Anti-Speed Limitation/3(VINP_ZoneSpdCrlMode_enum)
  [VTQD_GearActualPosn_enum] -> Anti-Speed Limitation/2(VTQD_GearActualPosn_enum)
  Anti-Speed Limitation/3(VVMC_MSASetSpd_kph) -> [VVMC_MSASetSpd_kph]
  Anti-Speed Limitation/2(VVMC_MSASpdCtrlMode_enum) -> [VVMC_MSASpdCtrlMode_enum]
  [VVMC_AntiSpdLimEn_flg] -> MSAActivationHandshake/10(VVMC_AntiSpdLimEn_flg)
  [VVMC_AntiSpdLimEn_flg] -> MSATorqueSourceDetermination/9(VVMC_AntiSpdLimEn_flg)
  [VVMC_CalMeterSpeed_kph] -> MSAActivationHandshake/11(VVMC_CalMeterSpeed_kph)
  Constant7/1 -> Switch5/3
  Switch5/1 -> [VVMC_ExtraMSACtrlSta_enum]  "VVMC_ExtraMSACtrlSta_enum"
  [VVMC_AntiSpdLimEn_flg] -> Switch5/2
  Constant6/1 -> Switch5/1
  [VVMC_ExtraMSACtrlSta_enum] -> VVMC_ExtraMSACtrlSta_enum/1

== system vmc/VMC/RDC Determination ==
  task_time_s : Inport
  VVMC_ActMaxSlideRate_pct : Inport  Port=2
  VTQD_AfterAvailableTqDemFr_Nm : Inport  Port=3
  VTQD_AfterAvailableTqDemRr_Nm : Inport  Port=4
  VINP_ESCActive_flg : Inport  Port=5
  VINP_SASAngle_Deg : Inport  Port=6
  VINP_LatAccel_Gps : Inport  Port=7
  VINP_VehSpeed_kph : Inport  Port=8
  VINP_YawRate_degps : Inport  Port=9
  VINP_RDCActive_enum : Inport  Port=10
  VINP_DIDGetDynoMode_flg : Inport  Port=11
  VVMC_CalibratedGyroY_Dps : Inport  Port=12
  VVMC_CalibratedAccY_G : Inport  Port=13
  Constant1 : Constant  Value=KVMC_RDCLatGSW_flg
  Constant83 : Constant  Value=KVMC_RDCYawRateSW_flg
  RWD : Subsystem
  Switch : Switch  Criteria=u2 > Threshold
  Switch1 : Switch  Criteria=u2 > Threshold
  VVMC_RWDRDCActive_enum : Outport
  VVMC_RDCEnSlideRate_pct : Outport  Port=2
  VVMC_ActStESCYaw_degps : Outport  Port=3
  wires:
  [VINP_YawRate_degps] -> RWD/9(VINP_YawRate_degps)
  VTQD_AfterAvailableTqDemFr_Nm/1 -> [VTQD_AfterAvailableTqDemFr_Nm]
  [VTQD_AfterAvailableTqDemRr_Nm] -> RWD/4(VTQD_AfterAvailableTqDemRr_Nm)
  [VINP_RDCActive_enum] -> RWD/10(VINP_RDCActive_enum)
  [VINP_VehSpeed_kph] -> RWD/8(VINP_VehSpeed_kph)
  [VVMC_RWDRDCActive_enum] -> VVMC_RWDRDCActive_enum/1
  [VINP_LatAccel_Gps] -> RWD/7(VINP_LatAccel_Gps)
  [VVMC_ActMaxSlideRate_pct] -> RWD/2(VVMC_ActMaxSlideRate_pct)
  [VINP_SASAngle_Deg] -> RWD/6(VINP_SASAngle_Deg)
  [task_time_s] -> RWD/1(task_time_s)
  [VTQD_AfterAvailableTqDemFr_Nm] -> RWD/3(VTQD_AfterAvailableTqDemFr_Nm)
  [VINP_ESCActive_flg] -> RWD/5(VINP_ESCActive_flg)
  VINP_RDCActive_enum/1 -> [VINP_RDCActive_enum]
  VINP_SASAngle_Deg/1 -> [VINP_SASAngle_Deg]
  VTQD_AfterAvailableTqDemRr_Nm/1 -> [VTQD_AfterAvailableTqDemRr_Nm]
  task_time_s/1 -> [task_time_s]
  VVMC_ActMaxSlideRate_pct/1 -> [VVMC_ActMaxSlideRate_pct]
  VINP_ESCActive_flg/1 -> [VINP_ESCActive_flg]
  VINP_VehSpeed_kph/1 -> [VINP_VehSpeed_kph]
  RWD/1(VVMC_RWDRDCActive_enum) -> [VVMC_RWDRDCActive_enum]
  RWD/2(VVMC_RDCEnSlideRate_pct) -> [VVMC_RDCEnSlideRate_pct]
  RWD/3(VVMC_ActStESCYaw_Dps) -> [VVMC_ActStESCYaw_degps]
  [VVMC_RDCEnSlideRate_pct] -> VVMC_RDCEnSlideRate_pct/1
  [VVMC_ActStESCYaw_degps] -> VVMC_ActStESCYaw_degps/1
  VINP_DIDGetDynoMode_flg/1 -> [VINP_DIDGetDynoMode_flg]
  [VINP_DIDGetDynoMode_flg] -> RWD/11(VINP_DIDGetDynoMode_flg)
  VVMC_CalibratedGyroY_Dps/1 -> Switch/1
  VINP_YawRate_degps/1 -> Switch/3
  Switch/1 -> [VINP_YawRate_degps]  "VINP_YawRate_degps"
  Constant83/1 -> Switch/2
  Constant1/1 -> Switch1/2
  VVMC_CalibratedAccY_G/1 -> Switch1/1
  VINP_LatAccel_Gps/1 -> Switch1/3
  Switch1/1 -> [VINP_LatAccel_Gps]  "VINP_LatAccel_Gps"
